simulink model "Ackeraman"  (R2019b)
settings: Solver=VariableStepAuto  StartTime=0.0  StopTime=simTime  RelTol=1e-3
values from neighbouring files (symbols this model uses):
  a0 = 1    [Ackerman_init.m]
  a1 = 4    [Ackerman_init.m]
  a2 = 3    [Ackerman_init.m]
  Change = 0    [Ackerman_init.m]
  k0 = 5    [Ackerman_init.m]
  k1 = place(Ad,bd,pd)    [Ackerman_init.m]
  k2 = place(Ac,bc,lambdatr')    [Ackerman_init.m]
  l = xlabel('Time (s)')    [Ackerman_init.m]
  pathType = 1    [Ackerman_init.m]
  phi0 = 0    [Ackerman_init.m]
  r = 2    [Ackerman_init.m]
  ref0 = [0 0]'    [Ackerman_init.m]
  refType = 1    [Ackerman_init.m]
  T = 0.3    [Ackerman_init.m]
  theta0 = pi    (= 3.14159265359)    [Ackerman_init.m]
  v0 = 2    [Ackerman_init.m]
  v_ref = 2    [Ackerman_init.m]
  x0 = 1    [Ackerman_init.m]
  y0 = 2    [Ackerman_init.m]
libraries: robotmobilelib x4
(part 4 of 4)

== matlab function Ackeraman/MATLAB Function6 ==
  data: c_old input; c output
function c  = fcn(c_old)

if c_old < 3
    c = c_old+1; 
else 
    c = 0;  
end

== matlab function Ackeraman/MATLAB Function7 ==
  data: ref_old input; delta_b input; ref_x1 output; v0 input; ref_x output; m parameter
function [ref_x1,ref_x] = fcn(ref_old, delta_b, v0, m)
delta = delta_b*3; 
a1 = m;
ref_old(2) = 0; 

ref_x1 = ref_old + [delta*v0*a1; v0*a1];

ref_x2 = ref_x1 + [delta*v0*a1; v0*a1];
ref_x = [ref_x1 ref_x2];

== matlab function Ackeraman/MATLAB Function8 ==
  data: tnref input; ref output; refType parameter; v_ref parameter
function ref = fcn(tnref,refType,v_ref)

if (refType == 1)
    ref = v_ref;
else
    ref = tnref(1,2);
    
end

== matlab function Ackeraman/MATLAB Function10 ==
  data: state input; v input; v_ref input; c input; pathType parameter; r parameter; a2 parameter; a1 parameter; a0 parameter; k0 parameter; l parameter; u output; w output; Change parameter; T parameter; refType parameter; k1 parameter
function [u,w] = MATLAB_Function5(state, v, v_ref, c ,pathType, r, a2, a1, a0, k0, l , Change, T, refType, k1)

x = state(1); y = state(2); theta = state(3); phi = state(4);
eta1 = v;
delta  = T;

if pathType == 1
    alpha = x^2+y^2 - r^2;
    dalpha = 2*v*(x*cos(theta) + y*sin(theta));
    ddalpha = (2*v^2*(l*cos(phi) + y*cos(theta)*sin(phi) - x*sin(phi)*sin(theta)))/(l*cos(phi));
    Lg1lfh2 = (2*eta1^2*(y*cos(theta) - x*sin(theta)))/(l*cos(phi)^2);
    Lf3     = -(2*eta1^3*sin(phi)^2*(x*cos(theta) + y*sin(theta)))/(l^2*cos(phi)^2);
else
    a       = 3; b       = 1.05*a;
    alpha = (x^2+y^2+a^2)^2-4*a^2*x^2-b^4; % defines the path
    dalpha = 4*v*y*sin(theta)*(a^2 + x^2 + y^2) + 4*v*x*cos(theta)*(- a^2 + x^2 + y^2);
    ddalpha = v*cos(theta)*(8*v*x^2*cos(theta) + 4*v*cos(theta)*(- a^2 + x^2 + y^2) + 8*v*x*y*sin(theta)) + v*sin(theta)*(4*v*sin(theta)*(a^2 + x^2 + y^2) + 8*v*y^2*sin(theta) + 8*v*x*y*cos(theta)) - (v*tan(phi)*(4*v*x*sin(theta)*(- a^2 + x^2 + y^2) - 4*v*y*cos(theta)*(a^2 + x^2 + y^2)))/l;
    Lg1lfh2 =  -(eta1*(tan(phi)^2 + 1)*(4*eta1*x*sin(theta)*(- a^2 + x^2 + y^2) - 4*eta1*y*cos(theta)*(a^2 + x^2 + y^2)))/l;
    Lf3     = -(4*eta1^3*(x^3*cos(theta)*sin(phi)^2 + y^3*sin(phi)^2*sin(theta) - 6*l^2*y*cos(phi)^2*sin(theta)^3 - 6*l^2*x*cos(phi)^2*cos(theta) - a^2*x*cos(theta)*sin(phi)^2 + a^2*y*sin(phi)^2*sin(theta) + x*y^2*cos(theta)*sin(phi)^2 + x^2*y*sin(phi)^2*sin(theta) - 6*l^2*y*cos(phi)^2*cos(theta)^2*sin(theta) - 6*a^2*l*cos(phi)*cos(theta)*sin(phi)*sin(theta) + 6*l*x^2*cos(phi)*cos(theta)*sin(phi)*sin(theta) - 6*l*y^2*cos(phi)*cos(theta)*sin(phi)*sin(theta) - 6*l*x*y*cos(phi)*cos(theta)^2*sin(phi) + 6*l*x*y*cos(phi)*sin(phi)*sin(theta)^2))/(l^2*cos(phi)^2);

end
if alpha < 1e-2 && Change == 1
    ref = 2*v_ref;
    L1 = exp(-k0*T); L2 = exp(-(k0)*T); 
else
    ref = v_ref;
    L1 = 0; L2 = 0; 
end


h = [alpha-delta*dalpha+delta^2/3*ddalpha;dalpha-delta/2*ddalpha;ddalpha];
u1 = -k0*(v-ref); 
v2 =  k1*h;

u = u1 ;
w = (Lg1lfh2)^(-1)*(-Lf3+v2);

== matlab function Ackeraman/MATLAB Function9 ==
  data: x output; state input; y output; theta output
function [x, y, theta] = fcn(state)

x = state(1);
y = state(2);
theta = state(3);
